simulink model "main"  (Simulink 4.00)
settings: Solver=ode45  StartTime=0.0  StopTime=10.0  RelTol=1e-3
settings Model: LastModifiedBy=User

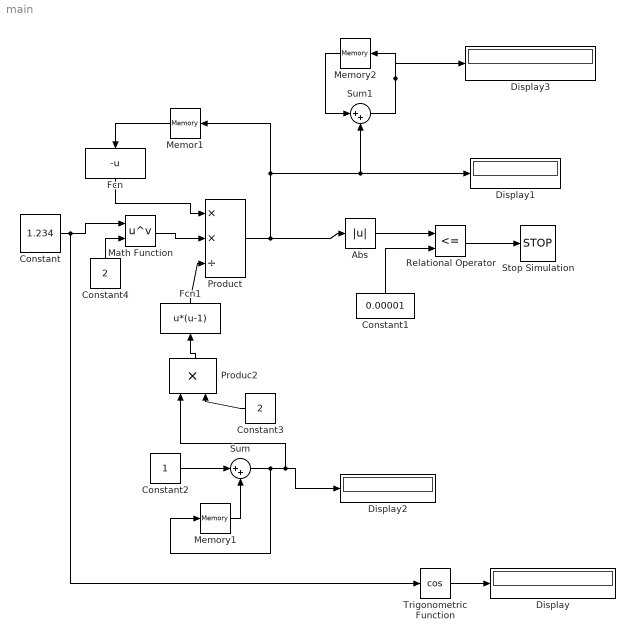
== system main ==
  Abs : Abs  SaturateOnIntegerOverflow=on
  Constant : Constant  Value=1.234
  Constant1 : Constant  Orientation=up  Value=0.00001
  Constant2 : Constant  Value=1
  Constant3 : Constant  Orientation=left  Value=2
  Constant4 : Constant  Orientation=up  Value=2
  Display{,1..3} (4 alike) : Display
      Display1 settings: Format=short
      Display2 settings: Format=short
  Fcn : Fcn  Orientation=down  Expr=-u
  Fcn1 : Fcn  Orientation=up  Expr=u*(u-1)
  Math Function : Math  Operator=pow  OutputSignalType=auto
  "Memor1 " : Memory  Orientation=left  X0=1  InheritSampleTime=off
      settings: RTWStateStorageClass=Auto
  Memory1 : Memory  X0=0  InheritSampleTime=off
      settings: RTWStateStorageClass=Auto
  Memory2 : Memory  Orientation=left  X0=1  InheritSampleTime=off
      settings: RTWStateStorageClass=Auto
  Produc2 : Product  Orientation=up  Inputs=2  Multiplication=Element-wise(.*)  SaturateOnIntegerOverflow=on
  Product : Product  Inputs=**/  Multiplication=Element-wise(.*)  SaturateOnIntegerOverflow=off
  Relational Operator : RelationalOperator  Operator=<=
  Stop Simulation : Stop
  Sum : Sum  Inputs=|++  SaturateOnIntegerOverflow=on
  Sum1 : Sum  Inputs=|++  SaturateOnIntegerOverflow=off
  Trigonometric Function : Trigonometry  Operator=cos  OutputSignalType=auto
  wires:
  Trigonometric Function/1 -> Display/1
  "Memor1 "/1 -> Fcn/1
  Product/1 -> "Memor1 "/1, Display1/1, Sum1/2, Abs/1
  Abs/1 -> Relational Operator/1
  Constant1/1 -> Relational Operator/2
  Relational Operator/1 -> Stop Simulation/1
  Constant2/1 -> Sum/1
  Memory1/1 -> Sum/2
  Sum/1 -> Memory1/1, Display2/1, Produc2/1
  Sum1/1 -> Memory2/1, Display3/1
  Memory2/1 -> Sum1/1
  Constant/1 -> Math Function/1, Trigonometric Function/1
  Constant4/1 -> Math Function/2
  Math Function/1 -> Product/2
  Fcn/1 -> Product/1
  Fcn1/1 -> Product/3
  Produc2/1 -> Fcn1/1
  Constant3/1 -> Produc2/2
